simulink model "plannerTest"  (R2023a)
settings: Solver=FixedStepDiscrete  StartTime=0.0  StopTime=inf  FixedStep=0.2  RelTol=1e-3
settings Model: Creator=mvelmuru  LastModifiedBy=vmano

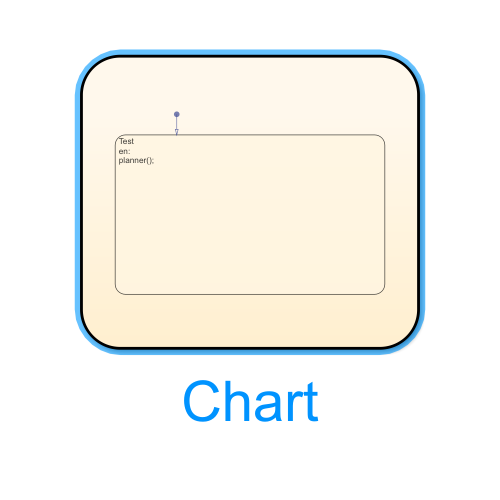
[thumbnail: Simulink's stored preview of the top-level diagram]
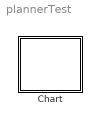
== system plannerTest ==
  Chart : Stateflow chart  TreatAsAtomicUnit=on

== stateflow chart plannerTest/Chart ==
  state Test
    en:
    coder.extrinsic('planner');
    startConfig = [0 0 0 0 0 0];
    goalConfig = [pi pi/2 0 0 0 0];
    planner([0.5, 0.5]);
  (default) -> Test
  data: goalConfig local; startConfig local
